simulink model "db4_10"  (R2018a)
settings: Solver=ode23  StartTime=0.0  StopTime=20  RelTol=1e-7  AbsTol=1e-9
values from neighbouring files (symbols this model uses):
  Kci = 1/Kti    (= 1)    [simulaciones.m]
  Kn = 0.6    [set_motor.m]
  Tci = 4*(Tpr+Tfi)    (= 0.03868)    [simulaciones.m]
libraries: simulink x2
settings Model: ExtModeTrigMode=oneshot  ExtModeArmWhenConnect=off  Creator=Administrador  LastModifiedBy=LAC-TELECOM-OLI-02
settings SolverCC: AutoScaleAbsTol=off
settings DataIOCC: SaveFormat=Array  SignalLoggingSaveFormat=ModelDataLogs
settings OptimizationCC: BlockReduction=off  BooleanDataType=off  ExpressionDepthLimit=2147483647  InitFltsAndDblsToZero=on  LifeSpan=inf
settings DebuggingCC: SaveWithParameterizedLinksMsg=none  UnderspecifiedInitializationDetection=Classic  MergeDetectMultiDrivingBlocksExec=none  SignalResolutionControl=TryResolveAllWithWarning  MultiTaskDSMMsg=warning  MultiTaskCondExecSysMsg=none  FcnCallInpInsideContextMsg=warning  StateNameClashWarn=warning  SFUnexpectedBacktrackingDiag=warning  SFNoUnconditionalDefaultTransitionDiag=warning  SFExecutionAtInitializationDiag=none
settings HardwareCC: ProdBitPerPointer=32  ProdBitPerSizeT=32  ProdBitPerPtrDiffT=32  ProdLargestAtomicFloat=None  ProdIntDivRoundTo=Undefined  ProdEndianess=Unspecified  ProdWordSize=32  ProdHWDeviceType=32-bit Generic  TargetUnknown=on
settings ModelReferenceCC: PropagateSignalLabelsOutOfModel=off
settings RTWCC: TemplateMakefile=grt_vc.tmf
settings CodeAppCC: StateflowObjectComments=on
settings GRTTargetCC: TargetLangStandard=C89/C90 (ANSI)  GeneratePreprocessorConditionals=Disable all  CombineOutputUpdateFcns=off  GRTInterface=on
settings ConfigComp: CovMetricSettings=dw  CovHtmlReporting=on  CovSaveCumulativeToWorkspaceVar=on  CovSaveSingleToWorkspaceVar=on  CovExternalEMLEnable=off

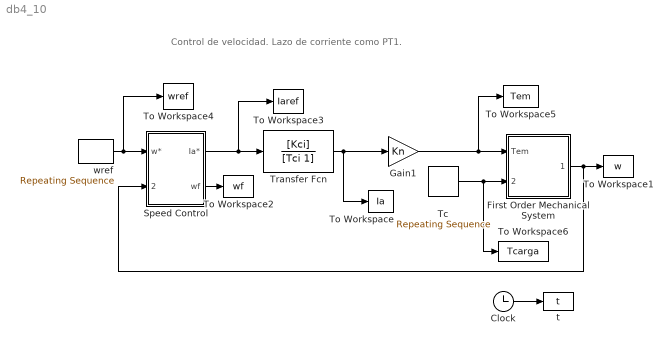
== system db4_10 ==
  note: Control de velocidad. Lazo de corriente como PT1.
  Clock : Clock
  First Order Mechanical System : Subsystem  mask(First Order Mechanical System){J=15, b=1.1, wor=0}
      mask prompts: J "Inertia [Kgm]:"; b "Friction Coeficient [Nm seg/rad]:"; wor "Speed Initial Condition [rad/sec]:"
      mask help:
      | This block solves the following differential equation:
      |
      | dW(t)/dt = - W(t)/J + (Tm - Load )/J
      | W(0)=W0
  Gain1 : Gain  Gain=Kn  SaturateOnIntegerOverflow=on  OutDataTypeStr=Inherit: Same as input  ParamDataTypeStr=Inherit: Same as input
  Speed Control : Subsystem  mask(Cascade Control for PMDCM (Controlled rectifier: PT1 or Dead Time)){d=on, Kpn=283.88, TIn=0.3135, Ktn=0.06, Tfn=0.008, Ian=319.6936}
      mask prompts: d "Zero Pre-compensation"; Kpn "Speed Proportional Gain:"; TIn "Speed Integral Gain:"; Ktn "Speed-sensor Proportional Gain:"; Tfn "Speed-sensor Integral Gain:"; Ian "Rated Armature Current [Amp]:"
      mask init:
      | if d==1
      | TIn_c=TIn;
      | else
      | TIn_c=0;
      | end
  Tc : simulink/Sources/Repeating Sequence  rep_seq_t=rep_seq_t  rep_seq_y=rep_seq_t
  To Workspace : ToWorkspace  VariableName=Ia  SampleTime=-1
  To Workspace1 : ToWorkspace  VariableName=w  SampleTime=-1
  To Workspace2 : ToWorkspace  VariableName=wf  SampleTime=-1
  To Workspace3 : ToWorkspace  VariableName=Iaref  SampleTime=-1
  To Workspace4 : ToWorkspace  VariableName=wref  SampleTime=-1
  To Workspace5 : ToWorkspace  VariableName=Tem  SampleTime=-1
  To Workspace6 : ToWorkspace  VariableName=Tcarga  SampleTime=-1
  Transfer Fcn : TransferFcn  Numerator=[Kci]  Denominator=[Tci 1]
  t : ToWorkspace  VariableName=t
      settings: MaxDataPoints=200000
  wref : simulink/Sources/Repeating Sequence  rep_seq_t=rep_seq_t  rep_seq_y=rep_seq_y
  wires:
  Speed Control/1(Ia*) -> Transfer Fcn/1, To Workspace3/1
  Transfer Fcn/1 -> Gain1/1, To Workspace/1
  wref/1 -> Speed Control/1(w*), To Workspace4/1
  Speed Control/2(wf) -> To Workspace2/1
  First Order Mechanical System/1(Wshaft) -> To Workspace1/1, Speed Control/2(Wshaft)
  Tc/1 -> First Order Mechanical System/2(TLoad), To Workspace6/1
  Gain1/1 -> First Order Mechanical System/1(Tem), To Workspace5/1
  Clock/1 -> t/1

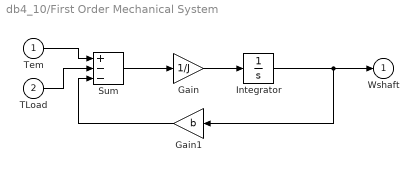
== system db4_10/First Order Mechanical System ==
  Tem : Inport
  TLoad : Inport  Port=2
  Gain : Gain  Gain=1/J  SaturateOnIntegerOverflow=on  OutDataTypeStr=Inherit: Same as input  ParamDataTypeStr=Inherit: Same as input
  Gain1 : Gain  Gain=b  SaturateOnIntegerOverflow=on  OutDataTypeStr=Inherit: Same as input  ParamDataTypeStr=Inherit: Same as input
  Integrator : Integrator  InitialCondition=wor
  Sum : Sum  Inputs=+--  SaturateOnIntegerOverflow=on  InputSameDT=on  OutDataTypeStr=Inherit: Same as first input
  Wshaft : Outport  InitialOutput=0
  wires:
  TLoad/1 -> Sum/2
  Tem/1 -> Sum/1
  Sum/1 -> Gain/1
  Gain/1 -> Integrator/1
  Gain1/1 -> Sum/3
  Integrator/1 -> Gain1/1, Wshaft/1

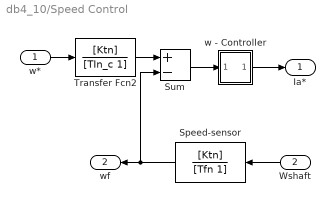
== system db4_10/Speed Control ==
  w* : Inport
  Wshaft : Inport  Port=2
  Speed-sensor : TransferFcn  Numerator=[Ktn]  Denominator=[Tfn 1]
  Sum : Sum  Inputs=+-  SaturateOnIntegerOverflow=on  InputSameDT=on  OutDataTypeStr=Inherit: Same as first input
  Transfer Fcn2 : TransferFcn  Numerator=[Ktn]  Denominator=[TIn_c 1]
  w - Controller : Subsystem  mask(PI Controller){P=Kpn, I=Kpn/TIn}
      mask prompts: P "Proportional:"; I "Integral:"
      mask help:
      | Enter expressions for proportional and  integral terms.
      | P+I/s
      mask Display: plot([0 0.001 5], [0 3 5])
  Ia* : Outport
  wf : Outport  Port=2
  wires:
  w - Controller/1(Out_1) -> Ia*/1
  Transfer Fcn2/1 -> Sum/1
  w*/1 -> Transfer Fcn2/1
  Wshaft/1 -> Speed-sensor/1
  Speed-sensor/1 -> Sum/2, wf/1
  Sum/1 -> w - Controller/1(In_1)

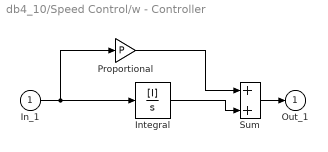
== system db4_10/Speed Control/w - Controller ==
  In_1 : Inport
  Integral : TransferFcn  Numerator=[I]  Denominator=[1 0]
  Proportional : Gain  Gain=P  SaturateOnIntegerOverflow=on  OutDataTypeStr=Inherit: Same as input  ParamDataTypeStr=Inherit: Same as input
  Sum : Sum  SaturateOnIntegerOverflow=on  InputSameDT=on  OutDataTypeStr=Inherit: Same as first input
  Out_1 : Outport
  wires:
  In_1/1 -> Proportional/1, Integral/1
  Sum/1 -> Out_1/1
  Integral/1 -> Sum/2
  Proportional/1 -> Sum/1
